simulink model "euler_to_rw_test"  (R2022b)
settings: Solver=VariableStepAuto  StartTime=0.0  StopTime=10.0  RelTol=1e-3
settings Model: Creator=Cal__  LastModifiedBy=Cal__

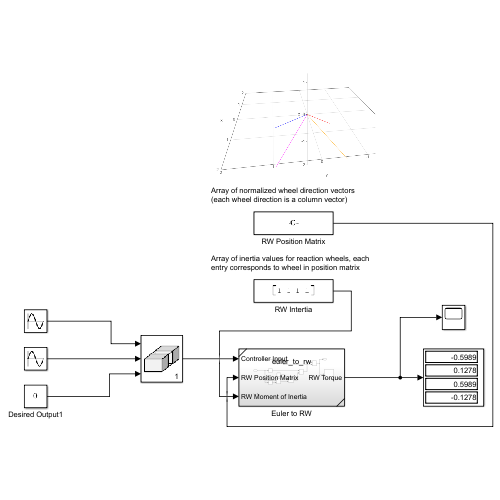
[thumbnail: Simulink's stored preview of the top-level diagram]
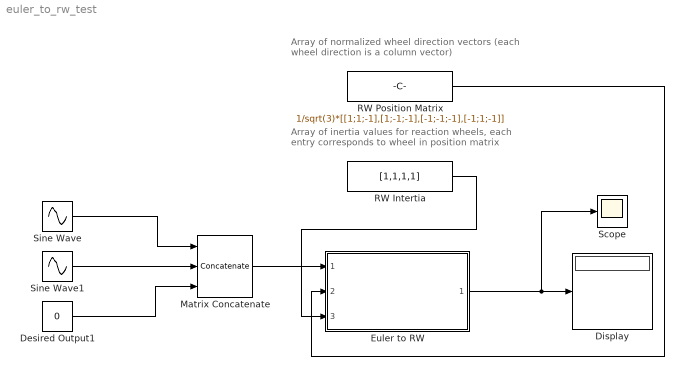
== system euler_to_rw_test ==
  note: Array of normalized wheel direction vectors (each wheel direction is a column vector)
  note: Array of inertia values for reaction wheels, each entry corresponds to wheel in position matrix
  Desired Output1 : Constant  Value=0
  Display : Display
  Euler to RW : Subsystem  ReferencedSubsystem=euler_to_rw
  Matrix Concatenate : Concatenate  NumInputs=3  Mode=Multidimensional array
  RW Intertia : Constant  Value=[1,1,1,1]
  RW Position Matrix : Constant  Value=1/sqrt(3)*[[1;1;-1],[1;-1;-1],[-1;-1;-1],[-1;1;-1]]
  Scope : Scope
  Sine Wave : Sin  SampleTime=0
  Sine Wave1 : Sin  Phase=pi/2  SampleTime=0
  wires:
  RW Intertia/1 -> Euler to RW/3
  RW Position Matrix/1 -> Euler to RW/2
  Euler to RW/1 -> Scope/1, Display/1
  Matrix Concatenate/1 -> Euler to RW/1
  Sine Wave/1 -> Matrix Concatenate/1
  Desired Output1/1 -> Matrix Concatenate/3
  Sine Wave1/1 -> Matrix Concatenate/2
